simulink model "vhf_control_unit_setup"  (R2024a)
settings: Solver=VariableStepAuto  StartTime=0.0  StopTime=10.0  RelTol=1e-3
undefined symbols (not defined in the file): alpha, g, Kp, M, N, Td, Ts
settings Model: Creator=Henrique Mesquita  LastModifiedBy=Henrique Mesquita

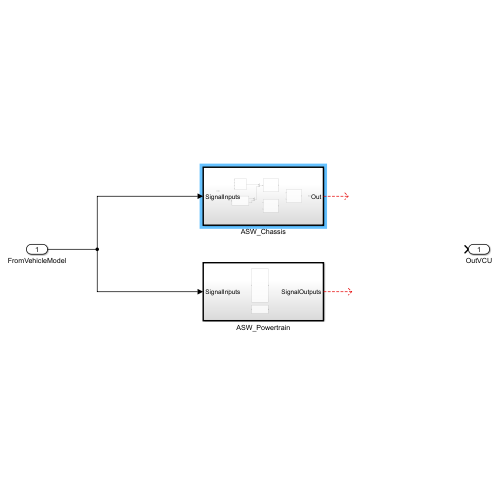
[thumbnail: Simulink's stored preview of the top-level diagram]
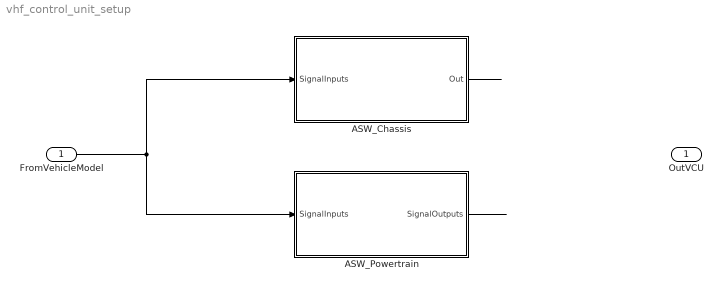
== system vhf_control_unit_setup ==
  FromVehicleModel : Inport
  ASW_Chassis : Subsystem  TreatAsAtomicUnit=on
  ASW_Powertrain : Subsystem  TreatAsAtomicUnit=on
  OutVCU : Outport
  wires:
  ASW_Chassis/1(Out) -> ?
  ASW_Powertrain/1(SignalOutputs) -> ?
  FromVehicleModel/1 -> ASW_Powertrain/1(SignalInputs), ASW_Chassis/1(SignalInputs)

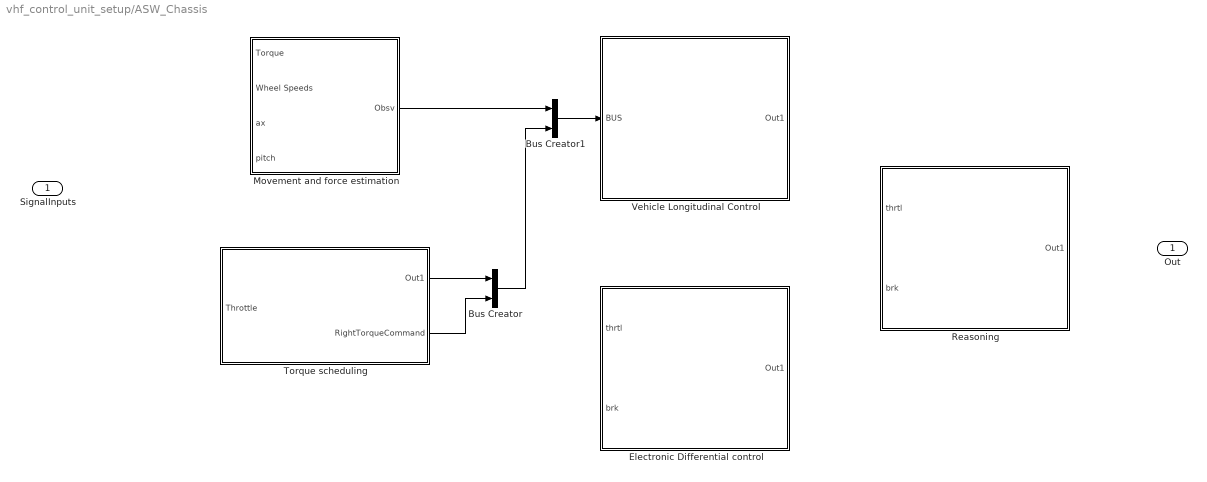
== system vhf_control_unit_setup/ASW_Chassis ==
  SignalInputs : Inport
  Bus Creator : BusCreator  Inputs=2
  Bus Creator1 : BusCreator  Inputs=2
  Electronic Differential control : Subsystem
  Movement and force estimation : Subsystem
  Reasoning : Subsystem
  Torque scheduling : Subsystem
  Vehicle Longitudinal Control : Subsystem
  Out : Outport
  wires:
  Torque scheduling/1(Out1) -> Bus Creator/1
  Torque scheduling/2(RightTorqueCommand) -> Bus Creator/2
  Bus Creator/1 -> Bus Creator1/2
  Movement and force estimation/1(Obsv) -> Bus Creator1/1
  Bus Creator1/1 -> Vehicle Longitudinal Control/1(BUS)

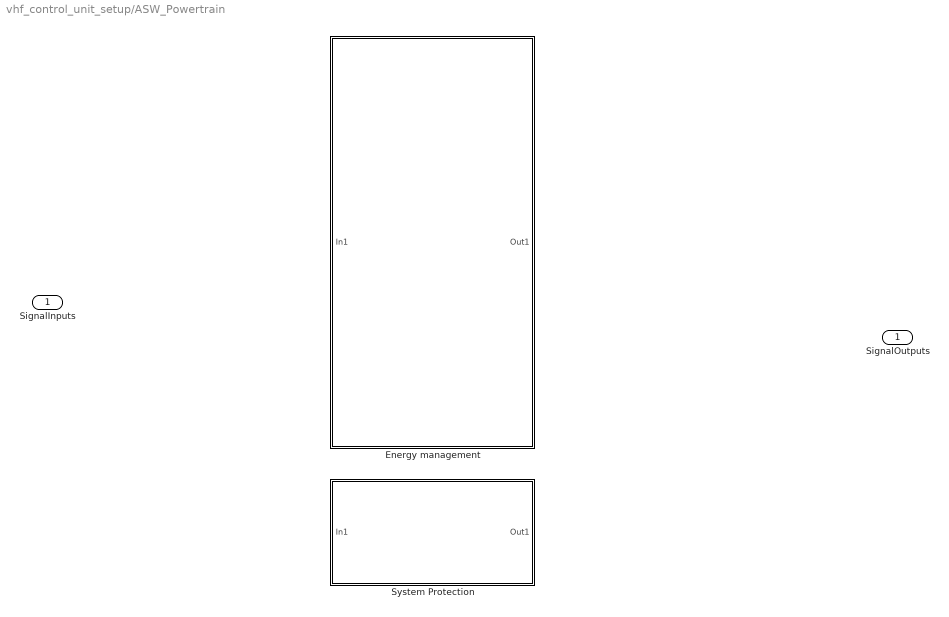
== system vhf_control_unit_setup/ASW_Powertrain ==
  SignalInputs : Inport
  Energy management : Subsystem
  System Protection : Subsystem
  SignalOutputs : Outport

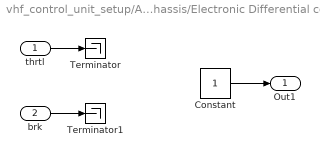
== system vhf_control_unit_setup/ASW_Chassis/Electronic Differential control ==
  thrtl : Inport
  brk : Inport  Port=2
  Constant : Constant
  Terminator : Terminator
  Terminator1 : Terminator
  Out1 : Outport
  wires:
  thrtl/1 -> Terminator/1
  brk/1 -> Terminator1/1
  Constant/1 -> Out1/1

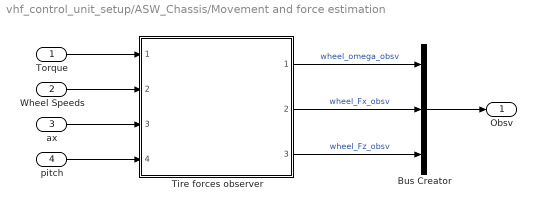
== system vhf_control_unit_setup/ASW_Chassis/Movement and force estimation ==
  Torque : Inport
  Wheel Speeds : Inport  Port=2
  ax : Inport  Port=3
  pitch : Inport  Port=4
  Bus Creator : BusCreator  Inputs=3
  Tire forces observer : Subsystem  ReferencedSubsystem=algebraic_PIO_observer
  Obsv : Outport
  wires:
  Tire forces observer/3 -> Bus Creator/3  "wheel_Fz_obsv"
  Tire forces observer/2 -> Bus Creator/2  "wheel_Fx_obsv"
  Tire forces observer/1 -> Bus Creator/1  "wheel_omega_obsv"
  Torque/1 -> Tire forces observer/1
  Wheel Speeds/1 -> Tire forces observer/2
  ax/1 -> Tire forces observer/3
  pitch/1 -> Tire forces observer/4
  Bus Creator/1 -> Obsv/1

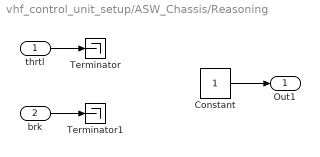
== system vhf_control_unit_setup/ASW_Chassis/Reasoning ==
  thrtl : Inport
  brk : Inport  Port=2
  Constant : Constant
  Terminator : Terminator
  Terminator1 : Terminator
  Out1 : Outport
  wires:
  thrtl/1 -> Terminator/1
  brk/1 -> Terminator1/1
  Constant/1 -> Out1/1

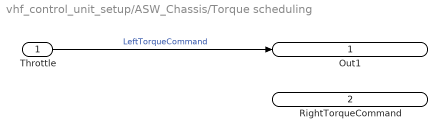
== system vhf_control_unit_setup/ASW_Chassis/Torque scheduling ==
  Throttle : Inport
  Out1 : Outport
  RightTorqueCommand : Outport  Port=2
  wires:
  Throttle/1 -> Out1/1  "LeftTorqueCommand"

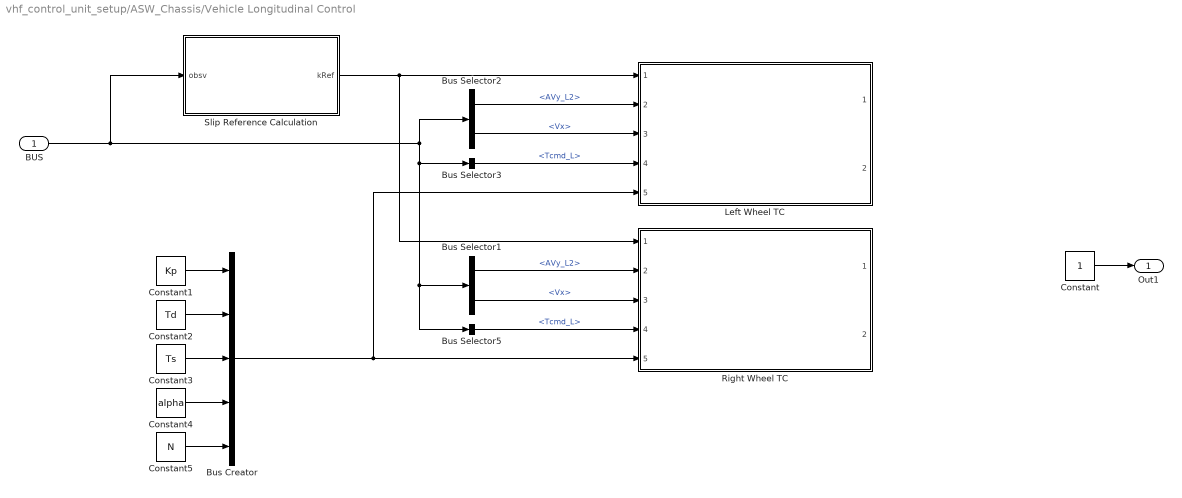
== system vhf_control_unit_setup/ASW_Chassis/Vehicle Longitudinal Control ==
  BUS : Inport
  Bus Creator : BusCreator  Inputs=5
  Bus Selector1 : BusSelector  OutputSignals=AVy_L2,Vx
  Bus Selector2 : BusSelector  OutputSignals=AVy_L2,Vx
  Bus Selector3 : BusSelector  OutputSignals=Tcmd_L
  Bus Selector5 : BusSelector  OutputSignals=Tcmd_L
  Constant : Constant
  Constant1 : Constant  Value=Kp
  Constant2 : Constant  Value=Td
  Constant3 : Constant  Value=Ts
  Constant4 : Constant  Value=alpha
  Constant5 : Constant  Value=N
  Left Wheel TC : Subsystem  ReferencedSubsystem=TractionControlMF
  Right Wheel TC : Subsystem  ReferencedSubsystem=TractionControlMF
  Slip Reference Calculation : Subsystem
  Out1 : Outport
  wires:
  BUS/1 -> Slip Reference Calculation/1(obsv), Bus Selector5/1, Bus Selector1/1, Bus Selector3/1, Bus Selector2/1
  Constant/1 -> Out1/1
  Constant1/1 -> Bus Creator/1
  Constant2/1 -> Bus Creator/2
  Constant3/1 -> Bus Creator/3
  Constant4/1 -> Bus Creator/4
  Constant5/1 -> Bus Creator/5
  Bus Creator/1 -> Left Wheel TC/5, Right Wheel TC/5
  Bus Selector1/1 -> Right Wheel TC/2  "<AVy_L2>"
  Bus Selector1/2 -> Right Wheel TC/3  "<Vx>"
  Bus Selector5/1 -> Right Wheel TC/4  "<Tcmd_L>"
  Bus Selector2/1 -> Left Wheel TC/2  "<AVy_L2>"
  Bus Selector2/2 -> Left Wheel TC/3  "<Vx>"
  Bus Selector3/1 -> Left Wheel TC/4  "<Tcmd_L>"
  Slip Reference Calculation/1(kRef) -> Right Wheel TC/1, Left Wheel TC/1

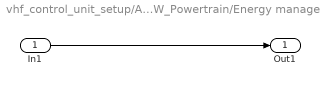
== system vhf_control_unit_setup/ASW_Powertrain/Energy management ==
  In1 : Inport
  Out1 : Outport
  wires:
  In1/1 -> Out1/1

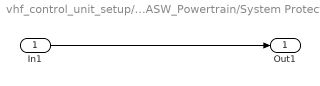
== system vhf_control_unit_setup/ASW_Powertrain/System Protection ==
  In1 : Inport
  Out1 : Outport
  wires:
  In1/1 -> Out1/1

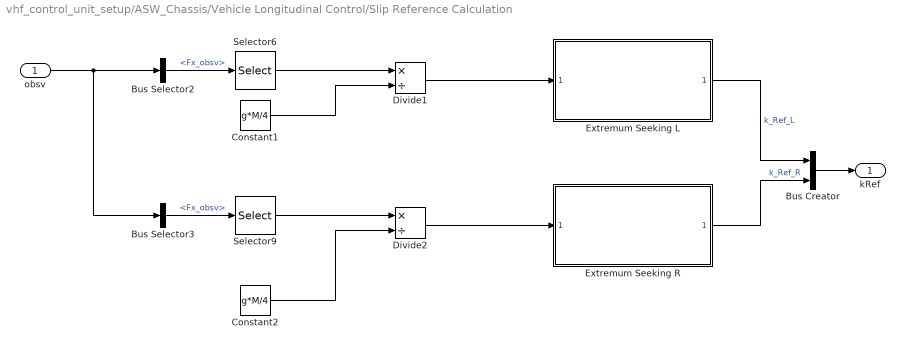
== system vhf_control_unit_setup/ASW_Chassis/Vehicle Longitudinal Control/Slip Reference Calculation ==
  obsv : Inport
  Bus Creator : BusCreator  Inputs=2
  Bus Selector2 : BusSelector  OutputSignals=Fx_obsv
  Bus Selector3 : BusSelector  OutputSignals=Fx_obsv
  Constant1 : Constant  Value=g*M/4
  Constant2 : Constant  Value=g*M/4
  Divide1 : Product  Inputs=*/
  Divide2 : Product  Inputs=*/
  Extremum Seeking L : Subsystem  ReferencedSubsystem=Extremum_Seeking_vx_gain
  Extremum Seeking R : Subsystem  ReferencedSubsystem=Extremum_Seeking_vx_gain
  Selector6 : Selector  InputPortWidth=4  IndexOptions=Index vector (dialog)  Indices=[3]  OutputSizes=1
  Selector9 : Selector  InputPortWidth=4  IndexOptions=Index vector (dialog)  Indices=[4]  OutputSizes=1
  kRef : Outport
  wires:
  Extremum Seeking L/1 -> Bus Creator/1  "k_Ref_L"
  Divide1/1 -> Extremum Seeking L/1
  Selector6/1 -> Divide1/1
  Constant1/1 -> Divide1/2
  Selector9/1 -> Divide2/1
  obsv/1 -> Bus Selector3/1, Bus Selector2/1
  Bus Selector2/1 -> Selector6/1  "<Fx_obsv>"
  Bus Selector3/1 -> Selector9/1  "<Fx_obsv>"
  Constant2/1 -> Divide2/2
  Divide2/1 -> Extremum Seeking R/1
  Extremum Seeking R/1 -> Bus Creator/2  "k_Ref_R"
  Bus Creator/1 -> kRef/1
